simulink model "simu"  (R2023a)
settings: Solver=VariableStepAuto  StartTime=0.0  StopTime=10.0  RelTol=1e-3
undefined symbols (not defined in the file): longueur
settings Model: Creator=daneydem1u  LastModifiedBy=daneydem1u

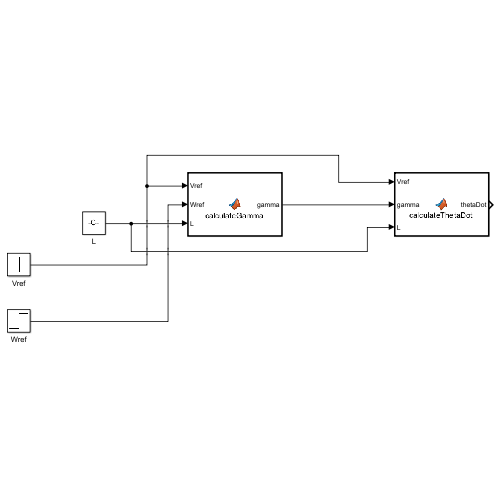
[thumbnail: Simulink's stored preview of the top-level diagram]
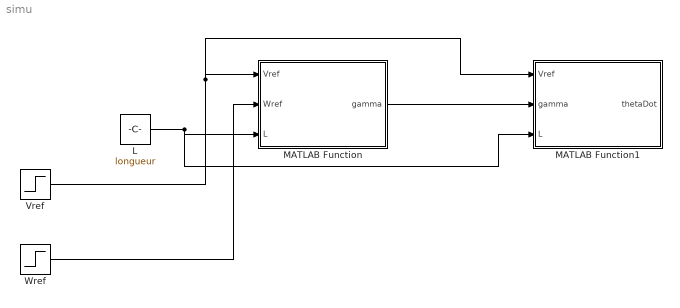
== system simu ==
  L : Constant  Value=longueur
  MATLAB Function : MATLAB Function  TreatAsAtomicUnit=on
  MATLAB Function1 : MATLAB Function  TreatAsAtomicUnit=on
  Vref : Step  SampleTime=0
  Wref : Step  SampleTime=0
  wires:
  L/1 -> MATLAB Function1/3(L), MATLAB Function/3(L)
  Vref/1 -> MATLAB Function1/1(Vref), MATLAB Function/1(Vref)
  Wref/1 -> MATLAB Function/2(Wref)
  MATLAB Function/1(gamma) -> MATLAB Function1/2(gamma)

== matlab function simu/MATLAB Function ==
  data: Vref input; gamma output; Wref input; L input
function gamma = calculateGamma(Vref, Wref, L)
    % Assurez-vous que Vref n'est pas zéro pour éviter une division par zéro
    if Vref == 0
        gamma = 0; % ou gérer autrement la condition de Vref zéro
    else
        gamma = atan((Wref * L) / Vref);
    end
end

== matlab function simu/MATLAB Function1 ==
  data: Vref input; thetaDot output; gamma input; L input
function thetaDot = calculateThetaDot(Vref, gamma, L)
    % Calcul de thetaDot
    thetaDot = Vref * tan(gamma) / L;
end
